simulink model "Simulink_model"  (R2021a)
settings: Solver=FixedStepAuto  StartTime=0.0  StopTime=1  FixedStep=0.01  RelTol=1e-3
settings Model: Creator=21694  LastModifiedBy=21694

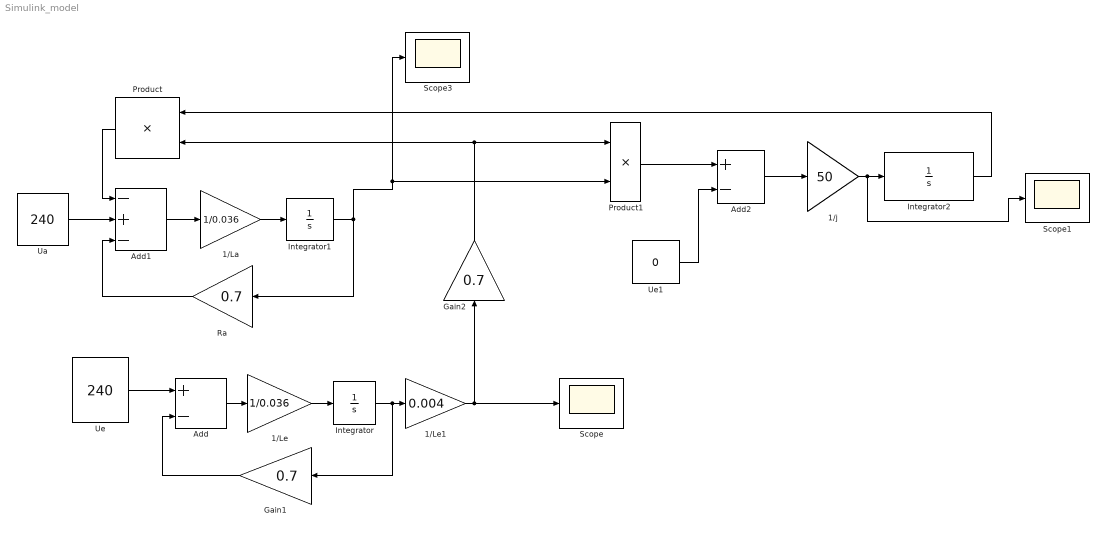
== system Simulink_model ==
  1/La : Gain  Gain=1/0.036
  1/Le : Gain  Gain=1/0.036
  1/Le1 : Gain  Gain=0.004
  1/j : Gain  Gain=50
  Add : Sum  Inputs=+-
  Add1 : Sum  Inputs=-+-
  Add2 : Sum  Inputs=+-
  Gain1 : Gain  Gain=0.7
  Gain2 : Gain  Gain=0.7
  Integrator : Integrator
  Integrator1 : Integrator
  Integrator2 : Integrator
  Product : Product
  Product1 : Product
  Ra : Gain  Gain=0.7
  Scope : Scope
  Scope1 : Scope
  Scope3 : Scope
  Ua : Constant  Value=240
  Ue : Constant  Value=240
  Ue1 : Constant  Value=0
  wires:
  Ue/1 -> Add/1
  Add/1 -> 1/Le/1
  1/Le/1 -> Integrator/1
  Integrator/1 -> Gain1/1, 1/Le1/1
  Gain1/1 -> Add/2
  Ua/1 -> Add1/2
  Add1/1 -> 1/La/1
  1/La/1 -> Integrator1/1
  Ra/1 -> Add1/3
  Integrator1/1 -> Scope3/1, Product1/2, Ra/1
  Product/1 -> Add1/1
  1/Le1/1 -> Gain2/1, Scope/1
  Product1/1 -> Add2/1
  Ue1/1 -> Add2/2
  Add2/1 -> 1/j/1
  Integrator2/1 -> Product/1
  Gain2/1 -> Product1/1, Product/2
  1/j/1 -> Scope1/1, Integrator2/1
